simulink model "inverted_pendulum"  (R2016b)
settings: Solver=VariableStepAuto  StartTime=0.0  StopTime=10  RelTol=1e-3
settings Model: Creator=Quy  LastModifiedBy=Quy

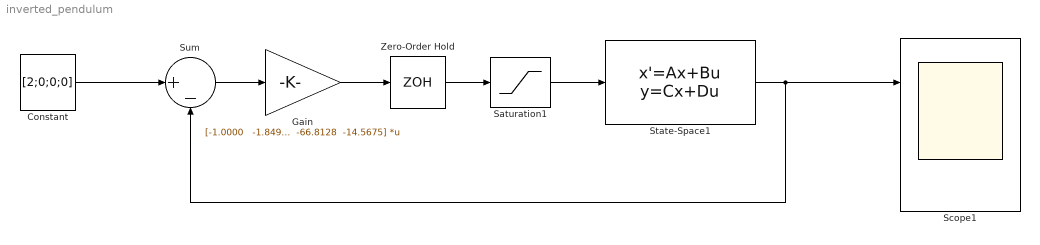
== system inverted_pendulum ==
  Constant : Constant  Value=[2;0;0;0]
  Gain : Gain  Gain="[-1.0000   -1.8497  -66.8128  -14.5675]"  Multiplication=Matrix(K*u) (u vector)
  Saturation1 : Saturate  UpperLimit=0.9  LowerLimit=-0.8
  Scope1 : Scope  NumInputPorts=2
  State-Space1 : StateSpace  A=|  B=|  C=eye(4)  D=[0; 0;0;0]  X0=[0; 0; 0; 1]
      A=|
      | [0    1.0000         0         0;
      |          0  -10.4100         0         0;
      |          0         0         0    1.0000;
      |          0    4.3111   36.7400   -0.6249]
      B=|
      | [0;
      |    51.2860;
      |          0;
      |   -21.0230]
  Sum : Sum  Inputs=|+-
  Zero-Order Hold : ZeroOrderHold  SampleTime=0.01
  wires:
  Gain/1 -> Zero-Order Hold/1
  Saturation1/1 -> State-Space1/1
  State-Space1/1 -> Sum/2, Scope1/1
  Constant/1 -> Sum/1
  Sum/1 -> Gain/1
  Zero-Order Hold/1 -> Saturation1/1
